simulink library "TCU_HPC"  (R2025b)
settings: Solver=VariableStepAuto  StartTime=0.0  StopTime=10.0  RelTol=1e-3
settings Model: Creator=joshu  LastModifiedBy=joshu

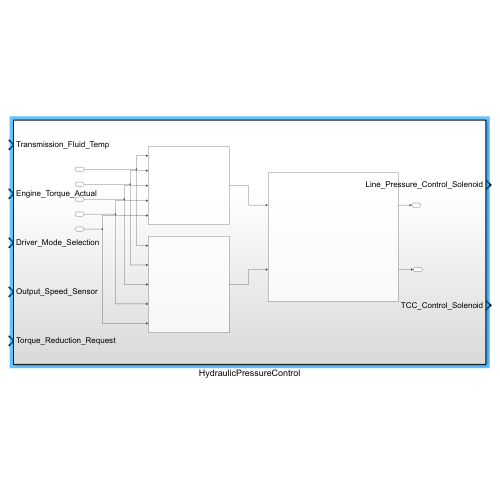
[thumbnail: Simulink's stored preview of the top-level diagram]
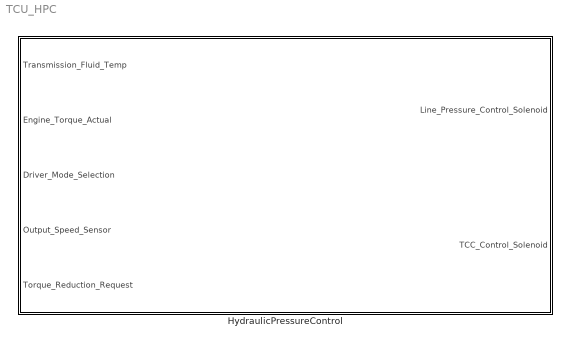
== system TCU_HPC ==
  HydraulicPressureControl : Subsystem

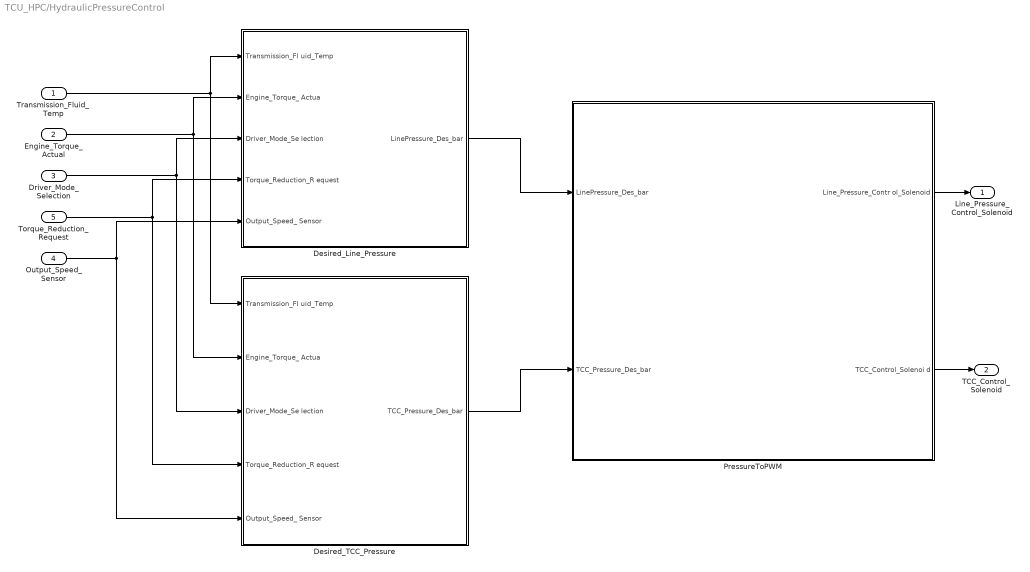
== system TCU_HPC/HydraulicPressureControl ==
  Transmission_Fluid_Temp : Inport
  Engine_Torque_Actual : Inport  Port=2
  "Driver_Mode_Selection " : Inport  Port=3
  Output_Speed_Sensor : Inport  Port=4
  Torque_Reduction_Request : Inport  Port=5
  Desired_Line_Pressure : Subsystem
  Desired_TCC_Pressure : Subsystem
  PressureToPWM : Subsystem
  Line_Pressure_Control_Solenoid : Outport
  TCC_Control_Solenoid : Outport  Port=2
  wires:
  Transmission_Fluid_Temp/1 -> Desired_TCC_Pressure/1(Transmission_Fl uid_Temp), Desired_Line_Pressure/1(Transmission_Fl uid_Temp)
  Engine_Torque_Actual/1 -> Desired_TCC_Pressure/2(Engine_Torque_ Actua), Desired_Line_Pressure/2(Engine_Torque_ Actua)
  "Driver_Mode_Selection "/1 -> Desired_TCC_Pressure/3("Driver_Mode_Se lection "), Desired_Line_Pressure/3("Driver_Mode_Se lection ")
  Torque_Reduction_Request/1 -> Desired_TCC_Pressure/4(Torque_Reduction_R equest), Desired_Line_Pressure/4(Torque_Reduction_R equest)
  Output_Speed_Sensor/1 -> Desired_Line_Pressure/5(Output_Speed_ Sensor), Desired_TCC_Pressure/5(Output_Speed_ Sensor)
  Desired_Line_Pressure/1(LinePressure_Des_bar) -> PressureToPWM/1(LinePressure_Des_bar)
  Desired_TCC_Pressure/1(TCC_Pressure_Des_bar) -> PressureToPWM/2(TCC_Pressure_Des_bar)
  PressureToPWM/1(Line_Pressure_Contr ol_Solenoid) -> Line_Pressure_Control_Solenoid/1
  PressureToPWM/2(TCC_Control_Solenoi d) -> TCC_Control_Solenoid/1

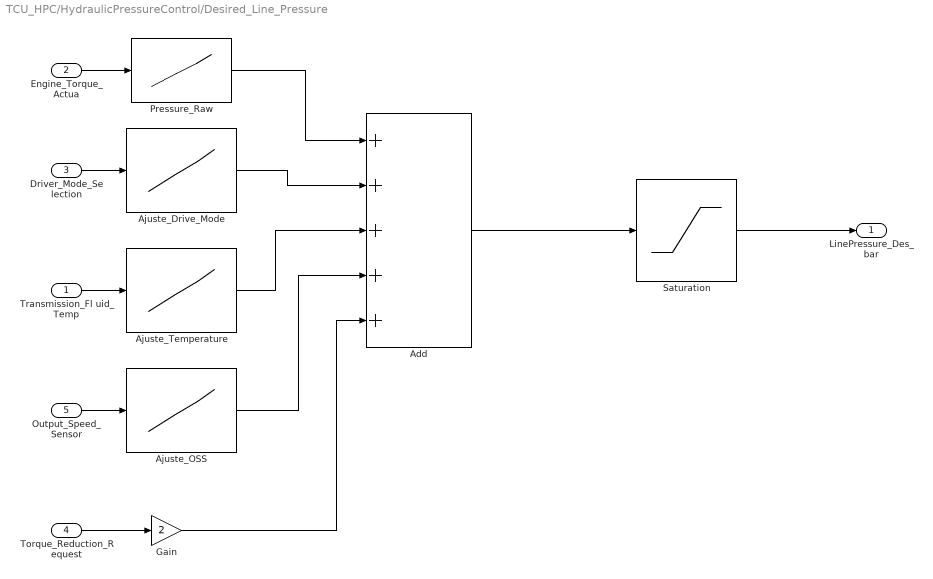
== system TCU_HPC/HydraulicPressureControl/Desired_Line_Pressure ==
  Transmission_Fl uid_Temp : Inport
  Engine_Torque_ Actua : Inport  Port=2
  "Driver_Mode_Se lection " : Inport  Port=3
  Torque_Reduction_R equest : Inport  Port=4
  Output_Speed_ Sensor : Inport  Port=5
  Add : Sum  Inputs=+++++
  Ajuste_Drive_Mode : Lookup_n-D  NumberOfTableDimensions=1  BreakpointsForDimension1=[0 1 2]  Table="[ -2.0  0.0  2.0 ]"  InternalRulePriority=Speed  RndMeth=Simplest
  Ajuste_OSS : Lookup_n-D  NumberOfTableDimensions=1  BreakpointsForDimension1="[    0   300   800  1500  2500  3500  4500 ]"  Table="[0.0  0.0  0.2  0.5  0.8  1.0  1.2 ]"  InternalRulePriority=Speed  RndMeth=Simplest
  Ajuste_Temperature : Lookup_n-D  NumberOfTableDimensions=1  BreakpointsForDimension1="[ -20    0   20   40   60   80  100  120 ]"  Table="[  3.0  2.0 1.5  0.5  0.0  0.0 0.5  1.0 ]"  InternalRulePriority=Speed  RndMeth=Simplest
  Gain : Gain  Gain=2
  Pressure_Raw : Lookup_n-D  NumberOfTableDimensions=1  BreakpointsForDimension1="[ 0   50  100  150  200  250  300  350 ]"  Table="[ 4.0 5.5  7.0  8.5 10.0 12.0 14.0 16.0 ]"  InternalRulePriority=Speed  RndMeth=Simplest
  Saturation : Saturate  UpperLimit=18  LowerLimit=4
  LinePressure_Des_bar : Outport
  wires:
  Engine_Torque_ Actua/1 -> Pressure_Raw/1
  "Driver_Mode_Se lection "/1 -> Ajuste_Drive_Mode/1
  Transmission_Fl uid_Temp/1 -> Ajuste_Temperature/1
  Output_Speed_ Sensor/1 -> Ajuste_OSS/1
  Torque_Reduction_R equest/1 -> Gain/1
  Pressure_Raw/1 -> Add/1
  Ajuste_Drive_Mode/1 -> Add/2
  Ajuste_Temperature/1 -> Add/3
  Ajuste_OSS/1 -> Add/4
  Gain/1 -> Add/5
  Add/1 -> Saturation/1
  Saturation/1 -> LinePressure_Des_bar/1

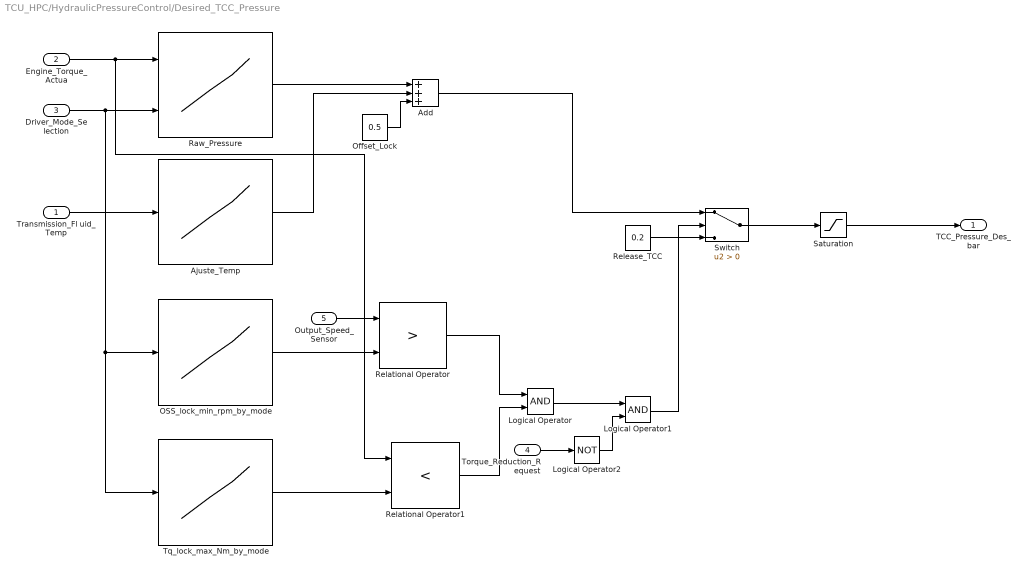
== system TCU_HPC/HydraulicPressureControl/Desired_TCC_Pressure ==
  Transmission_Fl uid_Temp : Inport
  Engine_Torque_ Actua : Inport  Port=2
  "Driver_Mode_Se lection " : Inport  Port=3
  Torque_Reduction_R equest : Inport  Port=4
  Output_Speed_ Sensor : Inport  Port=5
  Add : Sum  Inputs=+++
  Ajuste_Temp : Lookup_n-D  NumberOfTableDimensions=1  BreakpointsForDimension1="[ -20    0   20   40   60   80  100  120 ]"  Table="[ 0.2  0.2 0.1 0.0 0.0 0.0 0.1 0.2 ]"  InternalRulePriority=Speed  RndMeth=Simplest
  Logical Operator : Logic  AllPortsSameDT=off  OutDataTypeStr=boolean
  Logical Operator1 : Logic  AllPortsSameDT=off  OutDataTypeStr=boolean
  Logical Operator2 : Logic  Operator=NOT  AllPortsSameDT=off  OutDataTypeStr=boolean
  OSS_lock_min_rpm_by_mode : Lookup_n-D  NumberOfTableDimensions=1  BreakpointsForDimension1=[0 1 2]  Table="[ 1000  900  800 ]"  InternalRulePriority=Speed  RndMeth=Simplest
  Offset_Lock : Constant  Value=0.5
  Raw_Pressure : Lookup_n-D  BreakpointsForDimension1="[   0   50  100  150  200  250  300  350 ]"  BreakpointsForDimension2=[0 1 2]  Table=|  InternalRulePriority=Speed  RndMeth=Simplest
      | [
      |   0.4   0.5   0.6 ;
      |     0.6   0.7   0.8 ;
      |     0.8   0.9   1.0 ;
      |     1.0   1.1   1.2 ;
      |     1.2   1.3   1.4 ;
      |     1.4   1.5   1.6 ;
      |     1.6   1.7   1.8 ; 
      |     1.8   1.9   2.0 ]
      settings: InputPortMap=u0,u1
  Relational Operator : RelationalOperator  Operator=>  OutDataTypeStr=boolean  RndMeth=Simplest  InputSameDT=off
  Relational Operator1 : RelationalOperator  Operator=<  OutDataTypeStr=boolean  RndMeth=Simplest  InputSameDT=off
  Release_TCC : Constant  Value=0.2
  Saturation : Saturate  UpperLimit=8  LowerLimit=0
  Switch : Switch  Criteria=u2 > Threshold  SaturateOnIntegerOverflow=off  InputSameDT=off
  Tq_lock_max_Nm_by_mode : Lookup_n-D  NumberOfTableDimensions=1  BreakpointsForDimension1=[0 1 2]  Table="[ 180  220  260 ]"  InternalRulePriority=Speed  RndMeth=Simplest
  TCC_Pressure_Des_bar : Outport
  wires:
  Engine_Torque_ Actua/1 -> Relational Operator1/1, Raw_Pressure/1
  "Driver_Mode_Se lection "/1 -> Tq_lock_max_Nm_by_mode/1, OSS_lock_min_rpm_by_mode/1, Raw_Pressure/2
  Transmission_Fl uid_Temp/1 -> Ajuste_Temp/1
  Output_Speed_ Sensor/1 -> Relational Operator/1
  OSS_lock_min_rpm_by_mode/1 -> Relational Operator/2
  Tq_lock_max_Nm_by_mode/1 -> Relational Operator1/2
  Relational Operator/1 -> Logical Operator/1
  Relational Operator1/1 -> Logical Operator/2
  Logical Operator/1 -> Logical Operator1/1
  Torque_Reduction_R equest/1 -> Logical Operator2/1
  Logical Operator2/1 -> Logical Operator1/2
  Logical Operator1/1 -> Switch/2
  Ajuste_Temp/1 -> Add/2
  Raw_Pressure/1 -> Add/1
  Offset_Lock/1 -> Add/3
  Add/1 -> Switch/1
  Release_TCC/1 -> Switch/3
  Switch/1 -> Saturation/1
  Saturation/1 -> TCC_Pressure_Des_bar/1

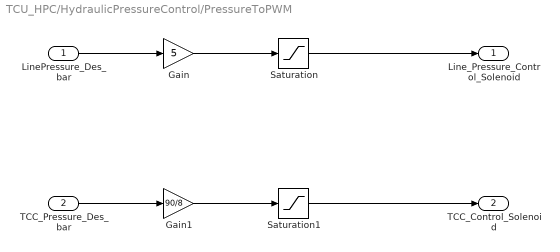
== system TCU_HPC/HydraulicPressureControl/PressureToPWM ==
  LinePressure_Des_bar : Inport
  TCC_Pressure_Des_bar : Inport  Port=2
  Gain : Gain  Gain=5
  Gain1 : Gain  Gain=90/8
  Saturation : Saturate  UpperLimit=100  LowerLimit=0
  Saturation1 : Saturate  UpperLimit=100  LowerLimit=0
  Line_Pressure_Contr ol_Solenoid : Outport
  TCC_Control_Solenoi d : Outport  Port=2
  wires:
  LinePressure_Des_bar/1 -> Gain/1
  Gain/1 -> Saturation/1
  Saturation/1 -> Line_Pressure_Contr ol_Solenoid/1
  Saturation1/1 -> TCC_Control_Solenoi d/1
  Gain1/1 -> Saturation1/1
  TCC_Pressure_Des_bar/1 -> Gain1/1
